simulink model "sampleModel204"  (R2021b)
settings: Solver=VariableStepAuto  StartTime=0.0  StopTime=10.0  RelTol=1e-3
undefined symbols (not defined in the file or in its folder): Newton, Raphson
libraries: simulink x6, slpidlib x3
settings Model: Creator=user  LastModifiedBy=user

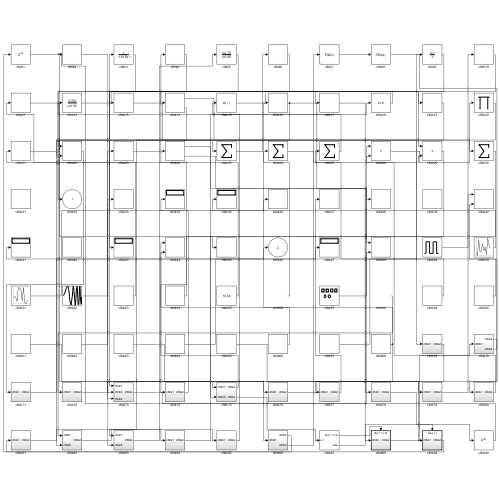
[thumbnail: Simulink's stored preview of the top-level diagram]
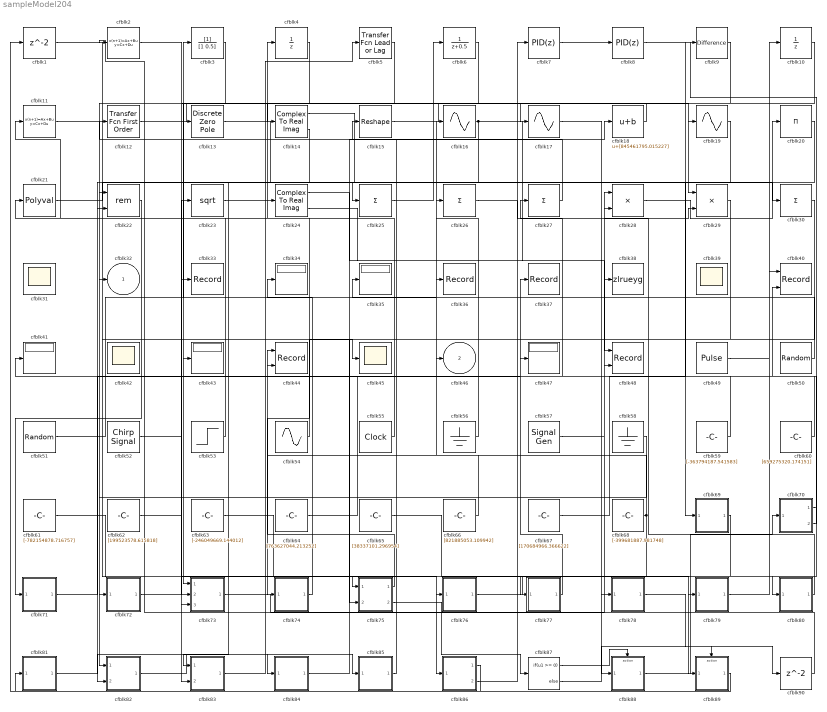
== system sampleModel204 ==
  cfblk1 : Delay  SampleTime=1
  cfblk10 : UnitDelay  HasFrameUpgradeWarning=on
  cfblk11 : DiscreteStateSpace
  cfblk12 : simulink/Discrete/Transfer Fcn First Order  PoleZ=0.95  ICPrevOutput=0.0  DoSatur=off
  cfblk13 : DiscreteZeroPole  Poles=[0 0.5]  Gain=1
  cfblk14 : ComplexToRealImag
  cfblk15 : Reshape
  cfblk16 : Sin  TimeSource=Use external signal  SampleTime=0
  cfblk17 : Sin  TimeSource=Use external signal  SampleTime=0
  cfblk18 : Bias  Bias=[845461795.015227]
  cfblk19 : Sin  TimeSource=Use external signal  SampleTime=0
  cfblk2 : DiscreteStateSpace
  cfblk20 : Product  Inputs=*
  cfblk21 : Polyval  Coefs=[ +2.081618890e-019, -1.441693666e-014, +4.719686976e-010, -8.536869453e-006, +1.621573104e-001, -8.087801117e+001 ]
  cfblk22 : Math  Operator=rem  SaturateOnIntegerOverflow=on
  cfblk23 : Sqrt  SaturateOnIntegerOverflow=on
  cfblk24 : ComplexToRealImag
  cfblk{25..27,30} (4 alike) : Sum  Inputs=+
  cfblk28 : Product  Inputs=**
  cfblk29 : Product
  cfblk3 : DiscreteFilter  SampleTime=1
  cfblk{31,39,42,45} (4 alike) : Scope
      cfblk31 settings: Floating=on
      cfblk39 settings: Floating=on
      cfblk42 settings: Floating=on
  cfblk33 : Record  FileSettingsInternal="{\"entries\":[{\"content\":{\"excelSettings\":{\"content\":{},\"type\":\"Streamout.ExcelSettings\"}},\"type\":\"Streamout.FileSettingStorage\",\"uuid\":\"4614327e-6d68-453b-8b22-e360a787c784\"}],\"packageUris\":[\"http://schema.mathworks.com/mf0/streamout_blocks/R2020a\"],\"version\":\"1.0\"}"  SignalsInternal="{\"entries\":[{\"content\":{\"signals\":[{\"content\":{\"blockPath\":[\"sampleModel204/cfblk33\"],\"channel\":[],\"dimensions\":[1],\"domain\":\"sampleModel204/cfblk33\",\"lineColor\":\"#d95319\",\"plots\":[1],\"port\":1,\"sid\":[\"\"],\"signalID\":7830,\"signalName\":\"cfblk62\"},\"type\":\"RecordBlkView.Signal\",\"uuid\":\"73eefb64-9ff5-4529-8fa5-b9cf3d236068\"}]},\"type\":\"RecordBlkView.InputSignals\",\"uuid\":\"d034e69d-cb16-4f24-b8c5-1be1b0cbd2c7\"}],\"packageUris\":[\"http://schema.mathworks.com/mf0/streamout_blocks/R2020a\"],\"version\":\"1.0\"}"  VisualizationBindings="{\"sparklinesplugin\":{\"info\":[{\"bindingParametersList\":[],\"subplotID\":1}]}}"
  cfblk{34..35,41,43,47} (5 alike) : Display
  cfblk36 : Record  FileSettingsInternal="{\"entries\":[{\"content\":{\"excelSettings\":{\"content\":{},\"type\":\"Streamout.ExcelSettings\"}},\"type\":\"Streamout.FileSettingStorage\",\"uuid\":\"273fffbf-c1de-4c74-a5f9-b15d57392e10\"}],\"packageUris\":[\"http://schema.mathworks.com/mf0/streamout_blocks/R2020a\"],\"version\":\"1.0\"}"  SignalsInternal="{\"entries\":[{\"content\":{\"signals\":[{\"content\":{\"blockPath\":[\"sampleModel204/cfblk36\"],\"channel\":[],\"dimensions\":[1],\"domain\":\"sampleModel204/cfblk36\",\"lineColor\":\"#77ac30\",\"plots\":[1],\"port\":1,\"sid\":[\"\"],\"signalID\":7842,\"signalName\":\"cfblk72\"},\"type\":\"RecordBlkView.Signal\",\"uuid\":\"099157b1-13d5-4ecc-8a56-fe1fbab54c4c\"}]},\"type\":\"RecordBlkView.InputSignals\",\"uuid\":\"1c521255-1461-4086-a910-e84576cd6c86\"}],\"packageUris\":[\"http://schema.mathworks.com/mf0/streamout_blocks/R2020a\"],\"version\":\"1.0\"}"  VisualizationBindings="{\"sparklinesplugin\":{\"info\":[{\"bindingParametersList\":[],\"subplotID\":1}]}}"
  cfblk37 : Record  FileSettingsInternal="{\"entries\":[{\"content\":{\"excelSettings\":{\"content\":{},\"type\":\"Streamout.ExcelSettings\"}},\"type\":\"Streamout.FileSettingStorage\",\"uuid\":\"e99169b0-8bbd-4adc-bc89-6a821c2eb76f\"}],\"packageUris\":[\"http://schema.mathworks.com/mf0/streamout_blocks/R2020a\"],\"version\":\"1.0\"}"  SignalsInternal="{\"entries\":[{\"content\":{\"signals\":[{\"content\":{\"blockPath\":[\"sampleModel204/cfblk37\"],\"channel\":[],\"dimensions\":[1],\"domain\":\"sampleModel204/cfblk37\",\"lineColor\":\"#b746ff\",\"plots\":[1],\"port\":1,\"sid\":[\"\"],\"signalID\":7806,\"signalName\":\"cfblk77\"},\"type\":\"RecordBlkView.Signal\",\"uuid\":\"b58d8220-4f6b-40a0-8985-ec7f20b7d218\"}]},\"type\":\"RecordBlkView.InputSignals\",\"uuid\":\"e264d71b-3544-4864-a4c8-23cd5ab33d92\"}],\"packageUris\":[\"http://schema.mathworks.com/mf0/streamout_blocks/R2020a\"],\"version\":\"1.0\"}"  VisualizationBindings="{\"sparklinesplugin\":{\"info\":[{\"bindingParametersList\":[],\"subplotID\":1}]}}"
  cfblk38 : ToWorkspace  VariableName=zlrueyg  SaveFormat=Timeseries  SampleTime=-1
  cfblk4 : UnitDelay  HasFrameUpgradeWarning=on
  cfblk40 : Record  FileSettingsInternal="{\"entries\":[{\"content\":{\"excelSettings\":{\"content\":{},\"type\":\"Streamout.ExcelSettings\"}},\"type\":\"Streamout.FileSettingStorage\",\"uuid\":\"cbd2d082-06ee-47d5-bd8d-4f1c9f04a451\"}],\"packageUris\":[\"http://schema.mathworks.com/mf0/streamout_blocks/R2020a\"],\"version\":\"1.0\"}"  Layout=[1 1]  SignalsInternal="{\"entries\":[{\"content\":{\"signals\":[{\"content\":{\"blockPath\":[\"sampleModel204/cfblk40\"],\"channel\":[],\"dimensions\":[1],\"domain\":\"sampleModel204/cfblk40\",\"lineColor\":\"#a2142f\",\"plots\":[1],\"port\":1,\"sid\":[\"\"],\"signalID\":7834,\"signalName\":\"cfblk79\"},\"type\":\"RecordBlkView.Signal\",\"uuid\":\"3b1cfed9-1420-47cd-881b-1f195950825b\"},{\"content\":{\"blockPath\":[\"sampleModel204/cfblk40\"],\"channel\":[],\"dimensions\":[1],\"domain\":\"sampleModel204/cfblk40\",\"lineColor\":\"#139fff\",\"plots\":[1],\"port\":2,\"sid\":[\"\"],\"signalID\":7838,\"signalName\":\"cfblk60\"},\"type\":\"RecordBlkView.Signal\",\"uuid\":\"e244ccd6-8439-40ac-a44e-c5ccb9b32657\"}]},\"type\":\"RecordBlkView.InputSignals\",\"uuid\":\"2346d5ee-e037-4b1f-a6c8-a6c1346a6bf9\"}],\"packageUris\":[\"http://schema.mathworks.com/mf0/streamout_blocks/R2020a\"],\"version\":\"1.0\"}"  VisualizationBindings="{\"xyplotplugin\":{\"info\":[{\"series\":[{\"bindingParametersList\":[{\"parameter\":\"X-Axis\",\"signalID\":7834,\"signalName\":\"cfblk79\"},{\"parameter\":\"Y-Axis\",\"signalID\":7838,\"signalName\":\"cfblk60\"}],\"seriesID\":54602}],\"subplotID\":1}]}}"  CompatibilityTag=XY
  cfblk44 : Record  FileSettingsInternal="{\"entries\":[{\"content\":{\"excelSettings\":{\"content\":{},\"type\":\"Streamout.ExcelSettings\"}},\"type\":\"Streamout.FileSettingStorage\",\"uuid\":\"00e44288-5fa3-4b54-8d93-aeff6a4aa51a\"}],\"packageUris\":[\"http://schema.mathworks.com/mf0/streamout_blocks/R2020a\"],\"version\":\"1.0\"}"  Layout=[1 1]  SignalsInternal="{\"entries\":[{\"content\":{\"signals\":[{\"content\":{\"blockPath\":[\"sampleModel204/cfblk44\"],\"channel\":[],\"dimensions\":[1],\"domain\":\"sampleModel204/cfblk44\",\"lineColor\":\"#a2142f\",\"plots\":[1],\"port\":1,\"sid\":[\"\"],\"signalID\":7810,\"signalName\":\"cfblk75:1\"},\"type\":\"RecordBlkView.Signal\",\"uuid\":\"d7162e4a-4f86-4723-8ae1-6ffcbfc36c1b\"},{\"content\":{\"blockPath\":[\"sampleModel204/cfblk44\"],\"channel\":[],\"dimensions\":[1],\"domain\":\"sampleModel204/cfblk44\",\"lineColor\":\"#139fff\",\"plots\":[1],\"port\":2,\"sid\":[\"\"],\"signalID\":7814,\"signalName\":\"cfblk68\"},\"type\":\"RecordBlkView.Signal\",\"uuid\":\"1ecf414f-d565-42b0-bbaf-fa39055f94a2\"}]},\"type\":\"RecordBlkView.InputSignals\",\"uuid\":\"04dcf0cd-3f78-46c2-9d2d-164729496477\"}],\"packageUris\":[\"http://schema.mathworks.com/mf0/streamout_blocks/R2020a\"],\"version\":\"1.0\"}"  VisualizationBindings="{\"xyplotplugin\":{\"info\":[{\"series\":[{\"bindingParametersList\":[{\"parameter\":\"X-Axis\",\"signalID\":7810,\"signalName\":\"cfblk75:1\"},{\"parameter\":\"Y-Axis\",\"signalID\":7814,\"signalName\":\"cfblk68\"}],\"seriesID\":60804}],\"subplotID\":1}]}}"  CompatibilityTag=XY
  cfblk48 : Record  FileSettingsInternal="{\"entries\":[{\"content\":{\"excelSettings\":{\"content\":{},\"type\":\"Streamout.ExcelSettings\"}},\"type\":\"Streamout.FileSettingStorage\",\"uuid\":\"2edb4c00-d95e-48a7-8cef-8a4f1b586e17\"}],\"packageUris\":[\"http://schema.mathworks.com/mf0/streamout_blocks/R2020a\"],\"version\":\"1.0\"}"  Layout=[1 1]  SignalsInternal="{\"entries\":[{\"content\":{\"signals\":[{\"content\":{\"blockPath\":[\"sampleModel204/cfblk48\"],\"channel\":[],\"dimensions\":[1],\"domain\":\"sampleModel204/cfblk48\",\"lineColor\":\"#a2142f\",\"plots\":[1],\"port\":1,\"sid\":[\"\"],\"signalID\":7818,\"signalName\":\"cfblk16\"},\"type\":\"RecordBlkView.Signal\",\"uuid\":\"7f00db83-bb6a-45eb-ae87-3391caf7e80c\"},{\"content\":{\"blockPath\":[\"sampleModel204/cfblk48\"],\"channel\":[],\"dimensions\":[1],\"domain\":\"sampleModel204/cfblk48\",\"lineColor\":\"#139fff\",\"plots\":[1],\"port\":2,\"sid\":[\"\"],\"signalID\":7822,\"signalName\":\"cfblk57\"},\"type\":\"RecordBlkView.Signal\",\"uuid\":\"5618d3fc-cfe5-48fd-a683-d16c70412c7c\"}]},\"type\":\"RecordBlkView.InputSignals\",\"uuid\":\"57fb8652-3949-4bb4-bbb9-316d4caebcdb\"}],\"packageUris\":[\"http://schema.mathworks.com/mf0/streamout_blocks/R2020a\"],\"version\":\"1.0\"}"  VisualizationBindings="{\"xyplotplugin\":{\"info\":[{\"series\":[{\"bindingParametersList\":[{\"parameter\":\"X-Axis\",\"signalID\":7818,\"signalName\":\"cfblk16\"},{\"parameter\":\"Y-Axis\",\"signalID\":7822,\"signalName\":\"cfblk57\"}],\"seriesID\":5655}],\"subplotID\":1}]}}"  CompatibilityTag=XY
  cfblk49 : DiscretePulseGenerator  PulseType=Time based  Amplitude=[-519499388.720965]  Period=[94571993.588733]  PulseWidth=5  PhaseDelay=[2.000000]
  cfblk5 : simulink/Discrete/Transfer Fcn Lead or Lag  PoleZ=0.95  ZeroZ=0.75  ICPrevOutput=0.0  ICPrevInput=0.0  DoSatur=off
      settings: SourceProductBaseCode=SL
  cfblk50 : UniformRandomNumber  Minimum=[-8292247236.991416]  Maximum=[3900943533.196655]  Seed=[55618585.000000]  SampleTime=0.1
  cfblk51 : RandomNumber  Mean=[79889.380075]  Variance=[28207.649343]  Seed=[592125441.000000]  SampleTime=0.1
  cfblk52 : simulink/Sources/Chirp Signal  f1=[32544062.382468]  T=[137921275.697866]  f2=[-910671732.089501]
  cfblk53 : Step  Time=[4.000000]  Before=[565151935.973644]  After=[622894084.092801]  SampleTime=0
  cfblk54 : Sin  Amplitude=[555177665.867173]  Bias=[-790741266.615498]  SampleTime=0
  cfblk55 : DigitalClock
  cfblk56 : Ground
  cfblk57 : SignalGenerator  Amplitude=[824030716.043719]
  cfblk58 : Ground
  cfblk59 : Constant  Value=[-363794187.541583]  SampleTime=1
  cfblk6 : DiscreteTransferFcn  SampleTime=1
  cfblk60 : Constant  Value=[659275320.174151]  SampleTime=1
  cfblk61 : Constant  Value=[-782154878.716757]  SampleTime=1
  cfblk62 : Constant  Value=[199523578.615818]  SampleTime=1
  cfblk63 : Constant  Value=[-246049669.144012]  SampleTime=1
  cfblk64 : Constant  Value=[763627044.213252]  SampleTime=1
  cfblk65 : Constant  Value=[38337101.296954]  SampleTime=1
  cfblk66 : Constant  Value=[821885053.109942]  SampleTime=1
  cfblk67 : Constant  Value=[170684966.366622]  SampleTime=1
  cfblk68 : Constant  Value=[-399681887.981748]  SampleTime=1
  cfblk69 : Subsystem
  cfblk7 : slpidlib/PID Controller  Controller=PID  Form=Parallel  TimeDomain=Discrete-time  UseExternalTs=off  SampleTime=1  IntegratorMethod=Forward Euler  FilterMethod=Forward Euler  ControllerParametersSource=internal  P=1  I=1  D=0  UseFilter=on  N=100  TunerSelectOption=Transfer Function Based (PID Tuner App)  InitialConditionSource=internal  InitialConditionForIntegrator=0  InitialConditionForFilter=0  DifferentiatorICPrevScaledInput=0  ExternalReset=none  TrackingMode=off  Kt=1  LimitOutput=off  SatLimitsSource=internal  UpperSaturationLimit=inf  LowerSaturationLimit=-inf  LinearizeAsGain=off  AntiWindupMode=none  Kb=1  POutMin=[]  POutMax=[]  IOutMin=[]  IOutMax=[]  DOutMin=[]  DOutMax=[]  NOutMin=[]  NOutMax=[]  SumOutMin=[]  SumOutMax=[]  SaturationOutMin=[]  SaturationOutMax=[]  PParamMin=[]  PParamMax=[]  IParamMin=[]  IParamMax=[]  DParamMin=[]  DParamMax=[]  NParamMin=[]  NParamMax=[]  KbParamMin=[]  KbParamMax=[]  KtParamMin=[]  KtParamMax=[]  KbOutMin=[]  KbOutMax=[]  KtOutMin=[]  KtOutMax=[]  IntegratorOutMin=[]  IntegratorOutMax=[]  FilterOutMin=[]  FilterOutMax=[]  SumI1OutMin=[]  SumI1OutMax=[]  SumI2OutMin=[]  SumI2OutMax=[]  SumI3OutMin=[]  SumI3OutMax=[]  SumI4OutMin=[]  SumI4OutMax=[]  SumDOutMin=[]  SumDOutMax=[]  DifferentiatorOutMin=[]  DifferentiatorOutMax=[]  FilterDiffOutCoefMin=[]  FilterDiffOutCoefMax=[]  ReciprocalOutMin=[]  ReciprocalOutMax=[]  SumDenOutMin=[]  SumDenOutMax=[]  SumNumOutMin=[]  SumNumOutMax=[]  DivideOutMin=[]  DivideOutMax=[]  UdiffTsProdOutMin=[]  UdiffTsProdOutMax=[]  NTsProdOutMin=[]  NTsProdOutMax=[]  UintegralTsProdOutMin=[]  UintegralTsProdOutMax=[]  UngainTsProdOutMin=[]  UngainTsProdOutMax=[]  IntegratorContinuousStateAttributes=''  IntegratorStateMustResolveToSignalObject=off  IntegratorRTWStateStorageClass=Auto  FilterContinuousStateAttributes=''  FilterStateMustResolveToSignalObject=off  FilterRTWStateStorageClass=Auto  ParallelPVariant=InternalParameters  IdealPVariant=Disabled  IVariant=InternalParameters  DVariant=InternalParameters  IntegratorVariant=Discrete  SatVariant=Disabled  AWVariant=Passthrough  PCopyVariant=Disabled  TRVariant=Disabled  FdbkBlocksVariant=Forward  IdealPFdbkVariant=Disabled  SatFdbkVariant=Disabled  DerivativeFilterVariant=ForwardEulerFilter  NVariant=InternalParameters  NCopyVariant=Disabled  FilterICVariant=InternalICsFilter  IntegratorICVariant=InternalICs  ExternalResetVariant=Disabled  TRSumVariant=Passthrough  SumFdbkVariant=Disabled  SumVariant=Sum_PID  TsampFilterVariant=InternalTs  TsampNgainVariant=Passthrough  TsampIntegralVariant=Passthrough  ExternalSaturationOutDataTypeStr=Inherit: Same as second input
  cfblk70 : Subsystem
  cfblk71 : Subsystem
  cfblk72 : Subsystem
  cfblk73 : Subsystem
  cfblk74 : Subsystem
  cfblk75 : Subsystem
  cfblk76 : Subsystem
  cfblk77 : Subsystem
  cfblk78 : Subsystem
  cfblk79 : Subsystem
  cfblk8 : slpidlib/PID Controller  Controller=PID  Form=Parallel  TimeDomain=Discrete-time  UseExternalTs=off  SampleTime=1  IntegratorMethod=Forward Euler  FilterMethod=Forward Euler  ControllerParametersSource=internal  P=1  I=1  D=0  UseFilter=on  N=100  TunerSelectOption=Transfer Function Based (PID Tuner App)  InitialConditionSource=internal  InitialConditionForIntegrator=0  InitialConditionForFilter=0  DifferentiatorICPrevScaledInput=0  ExternalReset=none  TrackingMode=off  Kt=1  LimitOutput=off  SatLimitsSource=internal  UpperSaturationLimit=inf  LowerSaturationLimit=-inf  LinearizeAsGain=off  AntiWindupMode=none  Kb=1  POutMin=[]  POutMax=[]  IOutMin=[]  IOutMax=[]  DOutMin=[]  DOutMax=[]  NOutMin=[]  NOutMax=[]  SumOutMin=[]  SumOutMax=[]  SaturationOutMin=[]  SaturationOutMax=[]  PParamMin=[]  PParamMax=[]  IParamMin=[]  IParamMax=[]  DParamMin=[]  DParamMax=[]  NParamMin=[]  NParamMax=[]  KbParamMin=[]  KbParamMax=[]  KtParamMin=[]  KtParamMax=[]  KbOutMin=[]  KbOutMax=[]  KtOutMin=[]  KtOutMax=[]  IntegratorOutMin=[]  IntegratorOutMax=[]  FilterOutMin=[]  FilterOutMax=[]  SumI1OutMin=[]  SumI1OutMax=[]  SumI2OutMin=[]  SumI2OutMax=[]  SumI3OutMin=[]  SumI3OutMax=[]  SumI4OutMin=[]  SumI4OutMax=[]  SumDOutMin=[]  SumDOutMax=[]  DifferentiatorOutMin=[]  DifferentiatorOutMax=[]  FilterDiffOutCoefMin=[]  FilterDiffOutCoefMax=[]  ReciprocalOutMin=[]  ReciprocalOutMax=[]  SumDenOutMin=[]  SumDenOutMax=[]  SumNumOutMin=[]  SumNumOutMax=[]  DivideOutMin=[]  DivideOutMax=[]  UdiffTsProdOutMin=[]  UdiffTsProdOutMax=[]  NTsProdOutMin=[]  NTsProdOutMax=[]  UintegralTsProdOutMin=[]  UintegralTsProdOutMax=[]  UngainTsProdOutMin=[]  UngainTsProdOutMax=[]  IntegratorContinuousStateAttributes=''  IntegratorStateMustResolveToSignalObject=off  IntegratorRTWStateStorageClass=Auto  FilterContinuousStateAttributes=''  FilterStateMustResolveToSignalObject=off  FilterRTWStateStorageClass=Auto  ParallelPVariant=InternalParameters  IdealPVariant=Disabled  IVariant=InternalParameters  DVariant=InternalParameters  IntegratorVariant=Discrete  SatVariant=Disabled  AWVariant=Passthrough  PCopyVariant=Disabled  TRVariant=Disabled  FdbkBlocksVariant=Forward  IdealPFdbkVariant=Disabled  SatFdbkVariant=Disabled  DerivativeFilterVariant=ForwardEulerFilter  NVariant=InternalParameters  NCopyVariant=Disabled  FilterICVariant=InternalICsFilter  IntegratorICVariant=InternalICs  ExternalResetVariant=Disabled  TRSumVariant=Passthrough  SumFdbkVariant=Disabled  SumVariant=Sum_PID  TsampFilterVariant=InternalTs  TsampNgainVariant=Passthrough  TsampIntegralVariant=Passthrough  ExternalSaturationOutDataTypeStr=Inherit: Same as second input
  cfblk80 : Subsystem
  cfblk81 : Subsystem
  cfblk82 : Subsystem
  cfblk83 : Subsystem
  cfblk84 : Subsystem
  cfblk85 : Subsystem
  cfblk86 : Subsystem
  cfblk87 : If  IfExpression=u1 >= 0  SampleTime=1
  cfblk88 : Subsystem  TreatAsAtomicUnit=on
  cfblk89 : Subsystem  TreatAsAtomicUnit=on
  cfblk9 : simulink/Discrete/Difference  ICPrevInput=0.0  OutMin=[]  OutMax=[]  OutDataTypeStr=Inherit: Inherit via back propagation  OutDataType=fixdt(1, 16)  OutScaling=2^-10  DoSatur=off
  cfblk90 : Delay  SampleTime=1
  cfblk32 : Outport
  cfblk46 : Outport  Port=2
  wires:
  cfblk1/1 -> cfblk75/1(cfblk1)
  cfblk22/1 -> cfblk71/1(cfblk1)
  cfblk27/1 -> cfblk2/1
  cfblk88/1(cfblk2) -> cfblk70/1(cfblk1)
  cfblk11/1 -> cfblk45/1
  cfblk73/1(cfblk2) -> cfblk28/1
  cfblk15/1 -> cfblk29/1
  cfblk17/1 -> cfblk78/1(cfblk1)
  cfblk82/1(cfblk2) -> cfblk84/1(cfblk1)
  cfblk65/1 -> cfblk89/1(cfblk1)
  cfblk63/1 -> cfblk86/1(cfblk1)
  cfblk7/1 -> cfblk8/1
  cfblk77/1(cfblk2) -> cfblk37/1
  cfblk86/1(cfblk2) -> cfblk1/1
  cfblk28/1 -> cfblk20/1
  cfblk75/1(cfblk2) -> cfblk44/1
  cfblk4/1 -> cfblk82/1(cfblk1)
  cfblk6/1 -> cfblk73/1(cfblk1)
  cfblk51/1 -> cfblk3/1
  cfblk16/1 -> cfblk48/1, cfblk83/1(cfblk1)
  cfblk21/1 -> cfblk30/1
  cfblk57/1 -> cfblk48/2
  cfblk13/1 -> cfblk25/1
  cfblk3/1 -> cfblk73/2(cfblk3)
  cfblk75/2(cfblk4) -> cfblk87/1
  cfblk2/1 -> cfblk19/1
  cfblk24/1 -> cfblk38/1
  cfblk8/1 -> cfblk80/1(cfblk1)
  cfblk19/1 -> cfblk82/2(cfblk5)
  cfblk50/1 -> cfblk35/1
  cfblk66/1 -> cfblk16/1
  cfblk86/2(cfblk4) -> cfblk7/1
  cfblk12/1 -> cfblk17/1
  cfblk74/1(cfblk2) -> cfblk34/1
  cfblk14/1 -> cfblk69/1(cfblk1)
  cfblk80/1(cfblk2) -> cfblk28/2
  cfblk14/2 -> cfblk32/1
  cfblk10/1 -> cfblk22/1
  cfblk5/1 -> cfblk43/1
  cfblk67/1 -> cfblk9/1
  cfblk85/1(cfblk2) -> cfblk15/1
  cfblk61/1 -> cfblk76/1(cfblk1)
  cfblk81/1(cfblk2) -> cfblk85/1(cfblk1)
  cfblk72/1(cfblk2) -> cfblk36/1
  cfblk76/1(cfblk2) -> cfblk79/1(cfblk1)
  cfblk68/1 -> cfblk44/2, cfblk83/2(cfblk5)
  cfblk24/2 -> cfblk88/1(cfblk1)
  cfblk62/1 -> cfblk33/1
  cfblk20/1 -> cfblk22/2
  cfblk64/1 -> cfblk46/1
  cfblk30/1 -> cfblk75/2(cfblk3)
  cfblk69/1(cfblk2) -> cfblk73/3(cfblk4)
  cfblk55/1 -> cfblk4/1
  cfblk83/1(cfblk2) -> cfblk5/1
  cfblk56/1 -> cfblk26/1
  cfblk59/1 -> cfblk27/1
  cfblk23/1 -> cfblk24/1
  cfblk54/1 -> cfblk21/1
  cfblk58/1 -> cfblk72/1(cfblk1)
  cfblk18/1 -> cfblk14/1
  cfblk26/1 -> cfblk29/2
  cfblk84/1(cfblk2) -> cfblk18/1
  cfblk52/1 -> cfblk23/1
  cfblk89/1(cfblk2) -> cfblk81/1(cfblk1)
  cfblk70/1(cfblk2) -> cfblk77/1(cfblk1)
  cfblk29/1 -> cfblk74/1(cfblk1)
  cfblk25/1 -> cfblk6/1
  cfblk70/2(cfblk4) -> cfblk41/1
  cfblk71/1(cfblk2) -> cfblk47/1
  cfblk9/1 -> cfblk13/1
  cfblk49/1 -> cfblk10/1
  cfblk79/1(cfblk2) -> cfblk40/1
  cfblk53/1 -> cfblk11/1
  cfblk60/1 -> cfblk40/2
  cfblk87/1 -> cfblk88/Action
  cfblk87/2 -> cfblk89/Action
  cfblk78/1(cfblk2) -> cfblk90/1
  cfblk90/1 -> cfblk12/1

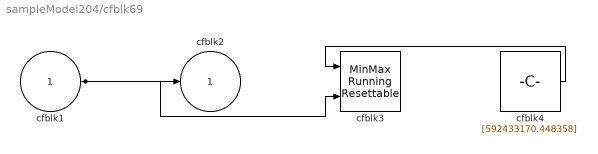
== system sampleModel204/cfblk69 ==
  cfblk1 : Inport
  cfblk3 : simulink/Math Operations/MinMax Running Resettable  Function=min  vinit=0.0
  cfblk4 : Constant  Value=[592433170.448358]  SampleTime=1
  cfblk2 : Outport
  wires:
  cfblk1/1 -> cfblk2/1, cfblk3/2
  cfblk4/1 -> cfblk3/1

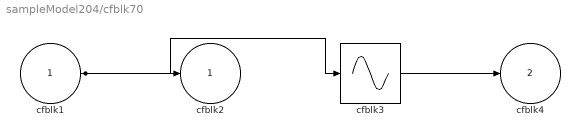
== system sampleModel204/cfblk70 ==
  cfblk1 : Inport
  cfblk3 : Sin  TimeSource=Use external signal  SampleTime=0
  cfblk2 : Outport
  cfblk4 : Outport  Port=2
  wires:
  cfblk1/1 -> cfblk3/1, cfblk2/1
  cfblk3/1 -> cfblk4/1

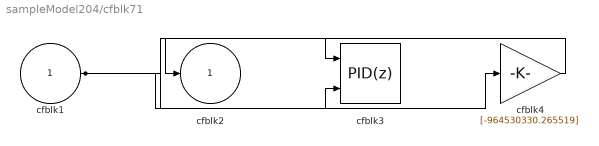
== system sampleModel204/cfblk71 ==
  cfblk1 : Inport
  cfblk3 : slpidlib/PID Controller (2DOF)  Controller=PID  Form=Parallel  TimeDomain=Discrete-time  UseExternalTs=off  SampleTime=1  IntegratorMethod=Forward Euler  FilterMethod=Forward Euler  ControllerParametersSource=internal  P=1  I=1  D=0  UseFilter=on  N=100  b=1  c=1  TunerSelectOption=Transfer Function Based (PID Tuner App)  InitialConditionSource=internal  InitialConditionForIntegrator=0  InitialConditionForFilter=0  DifferentiatorICPrevScaledInput=0  ExternalReset=none  TrackingMode=off  Kt=1  LimitOutput=off  SatLimitsSource=internal  UpperSaturationLimit=inf  LowerSaturationLimit=-inf  LinearizeAsGain=off  AntiWindupMode=none  Kb=1  POutMin=[]  POutMax=[]  IOutMin=[]  IOutMax=[]  DOutMin=[]  DOutMax=[]  NOutMin=[]  NOutMax=[]  bOutMin=[]  bOutMax=[]  cOutMin=[]  cOutMax=[]  SumOutMin=[]  SumOutMax=[]  SaturationOutMin=[]  SaturationOutMax=[]  PParamMin=[]  PParamMax=[]  IParamMin=[]  IParamMax=[]  DParamMin=[]  DParamMax=[]  NParamMin=[]  NParamMax=[]  bParamMin=[]  bParamMax=[]  cParamMin=[]  cParamMax=[]  KbParamMin=[]  KbParamMax=[]  KtParamMin=[]  KtParamMax=[]  KbOutMin=[]  KbOutMax=[]  KtOutMin=[]  KtOutMax=[]  IntegratorOutMin=[]  IntegratorOutMax=[]  FilterOutMin=[]  FilterOutMax=[]  SumI1OutMin=[]  SumI1OutMax=[]  SumI2OutMin=[]  SumI2OutMax=[]  SumI3OutMin=[]  SumI3OutMax=[]  SumI4OutMin=[]  SumI4OutMax=[]  SumDOutMin=[]  SumDOutMax=[]  Sum1OutMin=[]  Sum1OutMax=[]  Sum2OutMin=[]  Sum2OutMax=[]  Sum3OutMin=[]  Sum3OutMax=[]  DifferentiatorOutMin=[]  DifferentiatorOutMax=[]  FilterDiffOutCoefMin=[]  FilterDiffOutCoefMax=[]  ReciprocalOutMin=[]  ReciprocalOutMax=[]  SumDenOutMin=[]  SumDenOutMax=[]  SumNumOutMin=[]  SumNumOutMax=[]  DivideOutMin=[]  DivideOutMax=[]  UdiffTsProdOutMin=[]  UdiffTsProdOutMax=[]  NTsProdOutMin=[]  NTsProdOutMax=[]  UintegralTsProdOutMin=[]  UintegralTsProdOutMax=[]  UngainTsProdOutMin=[]  UngainTsProdOutMax=[]  IntegratorContinuousStateAttributes=''  IntegratorStateMustResolveToSignalObject=off  IntegratorRTWStateStorageClass=Auto  FilterContinuousStateAttributes=''  FilterStateMustResolveToSignalObject=off  FilterRTWStateStorageClass=Auto  ParallelPVariant=InternalParameters  IdealPVariant=Disabled  IVariant=InternalParameters  DVariant=InternalParameters  bVariant=InternalParameters  cVariant=InternalParameters  IntegratorVariant=Discrete  SatVariant=Disabled  AWVariant=Passthrough  PCopyVariant=Disabled  TRVariant=Disabled  FdbkBlocksVariant=Forward  IdealPFdbkVariant=Disabled  SatFdbkVariant=Disabled  DerivativeFilterVariant=ForwardEulerFilter  NVariant=InternalParameters  NCopyVariant=Disabled  FilterICVariant=InternalICsFilter  IntegratorICVariant=InternalICs  ExternalResetVariant=Disabled  TRSumVariant=Passthrough  SumFdbkVariant=Disabled  SumVariant=Sum_PID  TsampFilterVariant=InternalTs  TsampNgainVariant=Passthrough  TsampIntegralVariant=Passthrough  ExternalSaturationOutDataTypeStr=Inherit: Same as second input
      settings: SourceProductBaseCode=SL
  cfblk4 : Gain  Gain=[-964530330.265519]
  cfblk2 : Outport
  wires:
  cfblk4/1 -> cfblk2/1
  cfblk1/1 -> cfblk4/1, cfblk3/1, cfblk3/2

== system sampleModel204/cfblk72 ==
  cfblk1 : Inport
  cfblk3 : Signum
  cfblk2 : Outport
  wires:
  cfblk1/1 -> cfblk3/1
  cfblk3/1 -> cfblk2/1

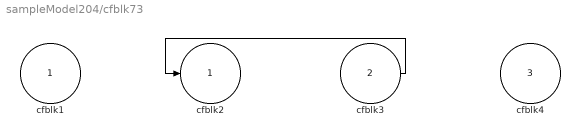
== system sampleModel204/cfblk73 ==
  cfblk1 : Inport
  cfblk3 : Inport  Port=2
  cfblk4 : Inport  Port=3
  cfblk2 : Outport
  wires:
  cfblk3/1 -> cfblk2/1

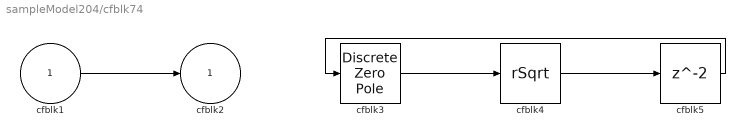
== system sampleModel204/cfblk74 ==
  cfblk1 : Inport
  cfblk3 : DiscreteZeroPole  Poles=[0 0.5]  Gain=1
  cfblk4 : Sqrt  Operator=rSqrt  AlgorithmType=Newton-Raphson  SaturateOnIntegerOverflow=on
  cfblk5 : Delay  SampleTime=1
  cfblk2 : Outport
  wires:
  cfblk3/1 -> cfblk4/1
  cfblk1/1 -> cfblk2/1
  cfblk4/1 -> cfblk5/1
  cfblk5/1 -> cfblk3/1

== system sampleModel204/cfblk75 ==
  cfblk1 : Inport
  cfblk3 : Inport  Port=2
  cfblk2 : Outport
  cfblk4 : Outport  Port=2
  wires:
  cfblk1/1 -> cfblk4/1
  cfblk3/1 -> cfblk2/1

== system sampleModel204/cfblk76 ==
  cfblk1 : Inport
  cfblk3 : Product  Inputs=**
  cfblk2 : Outport
  wires:
  cfblk1/1 -> cfblk3/1, cfblk3/2
  cfblk3/1 -> cfblk2/1

== system sampleModel204/cfblk77 ==
  cfblk1 : Inport
  cfblk3 : DotProduct  InputSameDT=on  OutDataTypeStr=Inherit: Inherit via internal rule
  cfblk2 : Outport
  wires:
  cfblk1/1 -> cfblk2/1, cfblk3/1, cfblk3/2

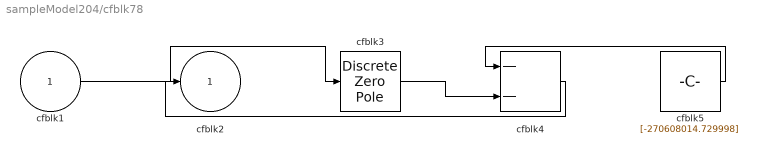
== system sampleModel204/cfblk78 ==
  cfblk1 : Inport
  cfblk3 : DiscreteZeroPole  Poles=[0 0.5]  Gain=1
  cfblk4 : Sum  Inputs=--
  cfblk5 : Constant  Value=[-270608014.729998]  SampleTime=1
  cfblk2 : Outport
  wires:
  cfblk1/1 -> cfblk3/1
  cfblk5/1 -> cfblk4/1
  cfblk3/1 -> cfblk4/2
  cfblk4/1 -> cfblk2/1

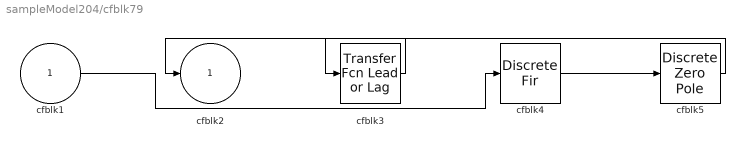
== system sampleModel204/cfblk79 ==
  cfblk1 : Inport
  cfblk3 : simulink/Discrete/Transfer Fcn Lead or Lag  PoleZ=0.95  ZeroZ=0.75  ICPrevOutput=0.0  ICPrevInput=0.0  DoSatur=off
      settings: SourceProductBaseCode=SL
  cfblk4 : DiscreteFir  SampleTime=1
  cfblk5 : DiscreteZeroPole  Poles=[0 0.5]  Gain=1
  cfblk2 : Outport
  wires:
  cfblk3/1 -> cfblk2/1
  cfblk1/1 -> cfblk4/1
  cfblk4/1 -> cfblk5/1
  cfblk5/1 -> cfblk3/1

== system sampleModel204/cfblk80 ==
  cfblk1 : Inport
  cfblk3 : DiscreteZeroPole  Poles=[0 0.5]  Gain=1
  cfblk2 : Outport
  wires:
  cfblk1/1 -> cfblk3/1
  cfblk3/1 -> cfblk2/1

== system sampleModel204/cfblk81 ==
  cfblk1 : Inport
  cfblk3 : Assignment  DiagnosticForDimensions=Warning  IndexOptions=Index vector (dialog)  Indices=1  OutputSizes=1
  cfblk2 : Outport
  wires:
  cfblk1/1 -> cfblk2/1, cfblk3/1, cfblk3/2

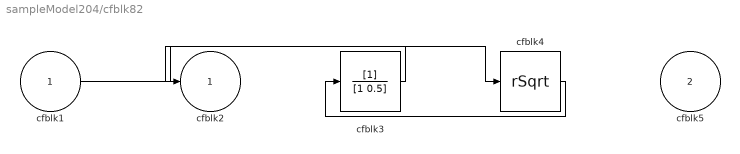
== system sampleModel204/cfblk82 ==
  cfblk1 : Inport
  cfblk5 : Inport  Port=2
  cfblk3 : DiscreteFilter  SampleTime=1
  cfblk4 : Sqrt  Operator=rSqrt  AlgorithmType=Newton-Raphson  SaturateOnIntegerOverflow=on
  cfblk2 : Outport
  wires:
  cfblk1/1 -> cfblk4/1
  cfblk4/1 -> cfblk3/1
  cfblk3/1 -> cfblk2/1

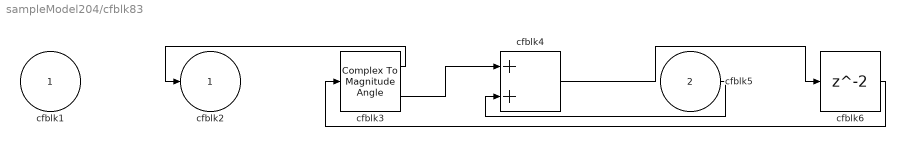
== system sampleModel204/cfblk83 ==
  cfblk1 : Inport
  cfblk5 : Inport  Port=2
  cfblk3 : ComplexToMagnitudeAngle
  cfblk4 : Sum
  cfblk6 : Delay  SampleTime=1
  cfblk2 : Outport
  wires:
  cfblk3/1 -> cfblk2/1
  cfblk3/2 -> cfblk4/1
  cfblk5/1 -> cfblk4/2
  cfblk4/1 -> cfblk6/1
  cfblk6/1 -> cfblk3/1

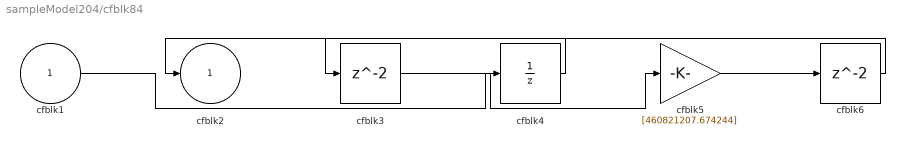
== system sampleModel204/cfblk84 ==
  cfblk1 : Inport
  cfblk3 : Delay  SampleTime=1
  cfblk4 : UnitDelay  HasFrameUpgradeWarning=on
  cfblk5 : Gain  Gain=[460821207.674244]
  cfblk6 : Delay  SampleTime=1
  cfblk2 : Outport
  wires:
  cfblk4/1 -> cfblk2/1
  cfblk3/1 -> cfblk5/1
  cfblk1/1 -> cfblk4/1
  cfblk5/1 -> cfblk6/1
  cfblk6/1 -> cfblk3/1

== system sampleModel204/cfblk85 ==
  cfblk1 : Inport
  cfblk3 : Sum  Inputs=-+
  cfblk2 : Outport
  wires:
  cfblk3/1 -> cfblk2/1
  cfblk1/1 -> cfblk3/1, cfblk3/2

== system sampleModel204/cfblk86 ==
  cfblk1 : Inport
  cfblk3 : Sqrt  SaturateOnIntegerOverflow=on
  cfblk2 : Outport
  cfblk4 : Outport  Port=2
  wires:
  cfblk1/1 -> cfblk2/1, cfblk3/1
  cfblk3/1 -> cfblk4/1

== system sampleModel204/cfblk88 ==
  cfblk1 : Inport
  Action Port : ActionPort  ActionPortLabel=if(u1 >= 0)
  cfblk3 : Sum  Inputs=|++
  cfblk2 : Outport
  wires:
  cfblk1/1 -> cfblk2/1, cfblk3/1, cfblk3/2

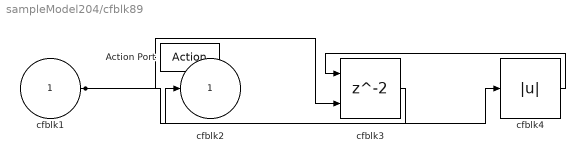
== system sampleModel204/cfblk89 ==
  cfblk1 : Inport
  Action Port : ActionPort  ActionPortLabel=else
  cfblk3 : Delay  ShowEnablePort=on
      settings: InputPortMap=u0,e6
  cfblk4 : Abs
  cfblk2 : Outport
  wires:
  cfblk3/1 -> cfblk2/1
  cfblk4/1 -> cfblk3/1
  cfblk1/1 -> cfblk3/2, cfblk4/1
